simulink model "AutoTranscontrol"  (R2020a)
settings: Solver=VariableStepAuto  StartTime=0.0  StopTime=10.0  RelTol=1e-3
values from neighbouring files (symbols this model uses):
  N20 = 0    [matlab_workspace.mat]
  Rfd = 3.23    [matlab_workspace.mat]
  rload0 = 40    [matlab_workspace.mat]
  rload2 = 0.02    [matlab_workspace.mat]
undefined symbols (not defined in the file or in its folder): EMAP, Kfactor, NE_VEC, speedratio, TH_VEC, Torkratio
settings Model: Creator=DELL  LastModifiedBy=DELL

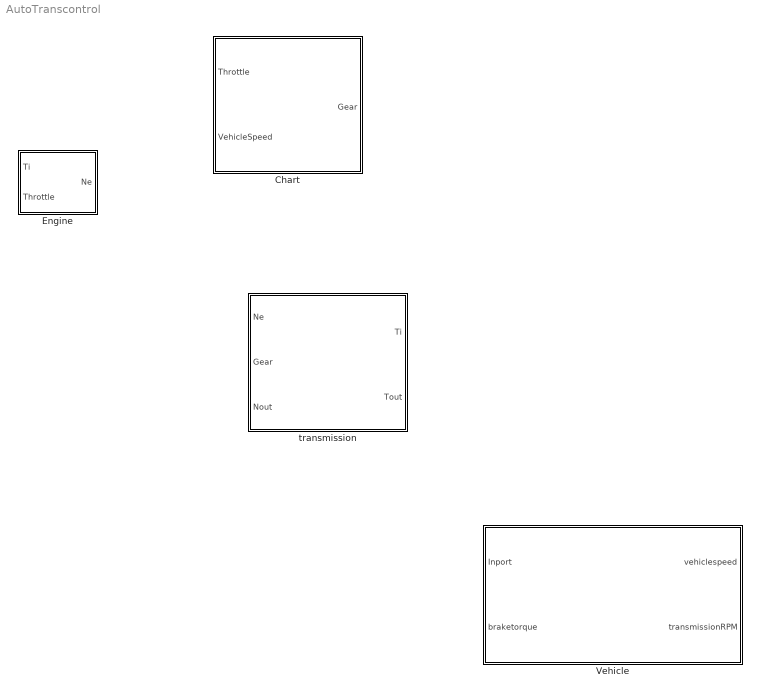
== system AutoTranscontrol ==
  Chart : Stateflow chart  TreatAsAtomicUnit=on
  Engine : Subsystem
  Vehicle : Subsystem
  transmission : Subsystem

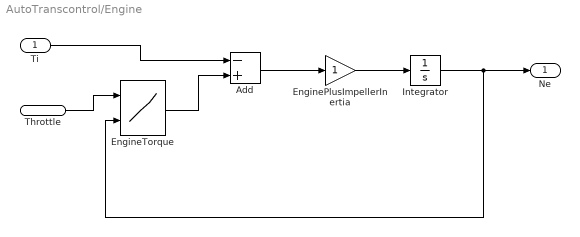
== system AutoTranscontrol/Engine ==
  Ti : Inport
  Throttle : Inport  Port=2
  Add : Sum  Inputs=-+
  EnginePlusImpellerInertia : Gain
  EngineTorque : Lookup_n-D  BreakpointsForDimension1=TH_VEC  BreakpointsForDimension2=NE_VEC  Table=EMAP  InputSameDT=on
  Integrator : Integrator  InitialCondition=1000  LimitOutput=on  UpperSaturationLimit=6000  LowerSaturationLimit=600
  Ne : Outport
  wires:
  EngineTorque/1 -> Add/2
  Add/1 -> EnginePlusImpellerInertia/1
  EnginePlusImpellerInertia/1 -> Integrator/1
  Integrator/1 -> Ne/1, EngineTorque/2
  Throttle/1 -> EngineTorque/1
  Ti/1 -> Add/1

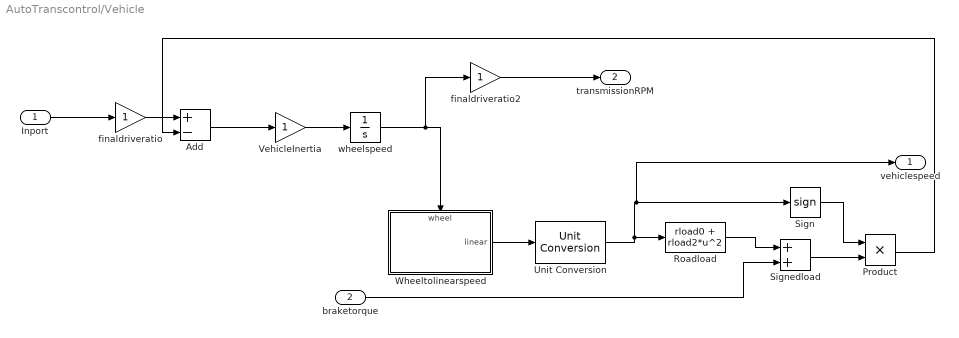
== system AutoTranscontrol/Vehicle ==
  Inport : Inport
  braketorque : Inport  Port=2
  Add : Sum  Inputs=+-
  Product : Product
  Roadload : Fcn  Expr=rload0 + rload2*u^2
  Sign : Signum
  Signedload : Sum
  Unit Conversion : UnitConversion
  VehicleInertia : Gain
  Wheeltolinearspeed : Subsystem
      settings: PortSchema="{\"entries\":[{\"content\":{\"sides\":[{\"content\":{\"connectorIds\":[]},\"type\":\"ConnectorPlacement.EquallySpacedRectSide\",\"uuid\":\"2d58122c-0a3c-46f5-9321-3a755b24d464\"},{\"content\":{\"connectorIds\":[\"Out1\"],\"side\":\"RIGHT\"},\"type\":\"ConnectorPlacement.EquallySpacedRectSide\",\"uuid\":\"52cb0b0a-ba8b-4201-a7b8-30d9f0796115\"},{\"content\":{\"connectorIds\":[\"In1\"],\"side\":\"TOP\"},\"type\":\"ConnectorPlacement.EquallySpacedRectSide\",\"uuid\":\"7f9df07b-7834-406d-9b53-00495da306c5\"}]},\"type\":\"ConnectorPlacement.EquallySpacedConnector\",\"uuid\":\"a8080389-0215-4d88-8d1d-d050e8a96295\"}],\"packageUris\":[\"http://schema.mathworks.com/mf0/Connector/19700101\"],\"version\":\"1.0\"}"
  finaldriveratio : Gain
  finaldriveratio2 : Gain
  wheelspeed : Integrator  InitialCondition=N20/Rfd
  vehiclespeed : Outport
  transmissionRPM : Outport  Port=2
  wires:
  wheelspeed/1 -> Wheeltolinearspeed/1(wheel), finaldriveratio2/1
  finaldriveratio/1 -> Add/1
  Inport/1 -> finaldriveratio/1
  Signedload/1 -> Product/2
  Sign/1 -> Product/1
  Wheeltolinearspeed/1(linear) -> Unit Conversion/1
  Add/1 -> VehicleInertia/1
  Roadload/1 -> Signedload/1
  Product/1 -> Add/2
  Unit Conversion/1 -> vehiclespeed/1, Sign/1, Roadload/1
  VehicleInertia/1 -> wheelspeed/1
  finaldriveratio2/1 -> transmissionRPM/1
  braketorque/1 -> Signedload/2

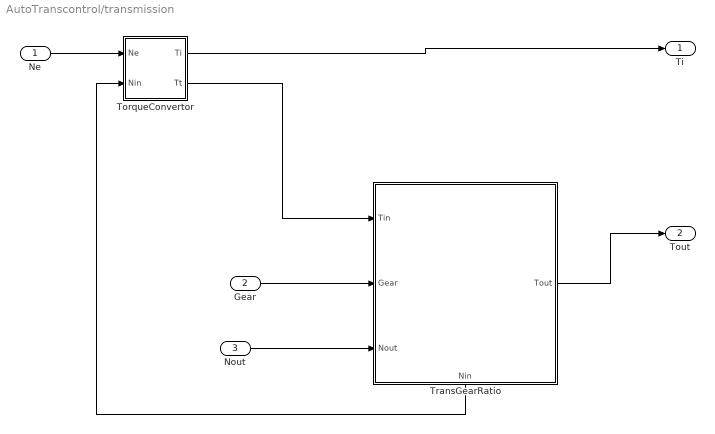
== system AutoTranscontrol/transmission ==
  Ne : Inport
  Gear : Inport  Port=2
  Nout : Inport  Port=3
  TorqueConvertor : Subsystem
  TransGearRatio : Subsystem
      settings: PortSchema="{\"entries\":[{\"content\":{\"sides\":[{\"content\":{\"connectorIds\":[\"In1\",\"In2\",\"In3\"]},\"type\":\"ConnectorPlacement.EquallySpacedRectSide\",\"uuid\":\"09106b39-6107-4922-852a-b097baa80348\"},{\"content\":{\"connectorIds\":[\"Out1\"],\"side\":\"RIGHT\"},\"type\":\"ConnectorPlacement.EquallySpacedRectSide\",\"uuid\":\"a36499d8-4a64-4af8-b2a6-947dde178184\"},{\"content\":{\"connectorIds\":[],\"side\":\"TOP\"},\"type\":\"ConnectorPlacement.EquallySpacedRectSide\",\"uuid\":\"0760f0ab-9b3f-4350-8835-7d8dce412455\"},{\"content\":{\"connectorIds\":[\"Out2\"],\"side\":\"BOTTOM\"},\"type\":\"ConnectorPlacement.EquallySpacedRectSide\",\"uuid\":\"6f573f33-3036-4647-848b-7112eae27f22\"}]},\"type\":\"ConnectorPlacement.EquallySpacedConnector\",\"uuid\":\"7220d938-930b-4b39-bb4b-0064243f33d7\"}],\"packageUris\":[\"http://schema.mathworks.com/mf0/Connector/19700101\"],\"version\":\"1.0\"}"
  Ti : Outport
  Tout : Outport  Port=2
  wires:
  Gear/1 -> TransGearRatio/2(Gear)
  Ne/1 -> TorqueConvertor/1(Ne)
  TorqueConvertor/1(Ti) -> Ti/1
  Nout/1 -> TransGearRatio/3(Nout)
  TransGearRatio/1(Tout) -> Tout/1
  TransGearRatio/2(Nin) -> TorqueConvertor/2(Nin)
  TorqueConvertor/2(Tt) -> TransGearRatio/1(Tin)

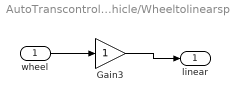
== system AutoTranscontrol/Vehicle/Wheeltolinearspeed ==
  wheel : Inport
  Gain3 : Gain
  linear : Outport
  wires:
  Gain3/1 -> linear/1
  wheel/1 -> Gain3/1

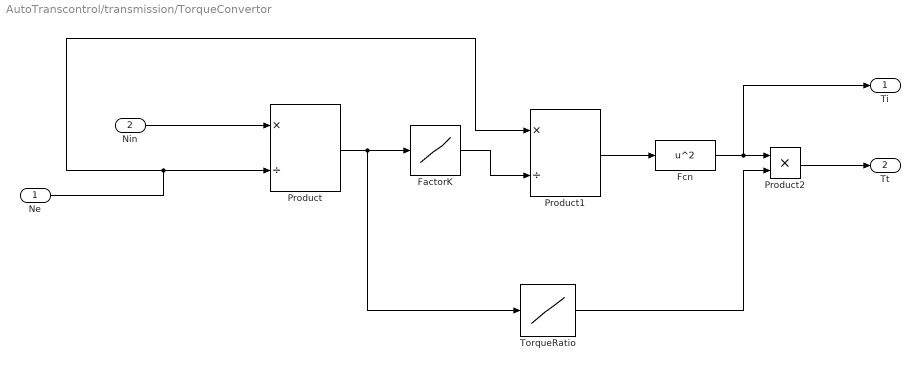
== system AutoTranscontrol/transmission/TorqueConvertor ==
  Ne : Inport
  Nin : Inport  Port=2
  FactorK : Lookup_n-D  NumberOfTableDimensions=1  BreakpointsForDimension1=speedratio  Table=Kfactor  SaturateOnIntegerOverflow=on  InputSameDT=on
  Fcn : Fcn  Expr=u^2
  Product : Product  Inputs=*/
  Product1 : Product  Inputs=*/
  Product2 : Product
  TorqueRatio : Lookup_n-D  NumberOfTableDimensions=1  BreakpointsForDimension1=speedratio  Table=Torkratio  SaturateOnIntegerOverflow=on  InputSameDT=on
  Ti : Outport
  Tt : Outport  Port=2
  wires:
  Product/1 -> TorqueRatio/1, FactorK/1
  Ne/1 -> Product1/1, Product/2
  FactorK/1 -> Product1/2
  Fcn/1 -> Ti/1, Product2/1
  Nin/1 -> Product/1
  Product2/1 -> Tt/1
  TorqueRatio/1 -> Product2/2
  Product1/1 -> Fcn/1

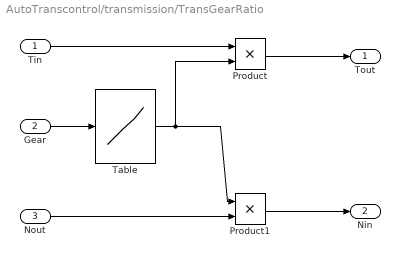
== system AutoTranscontrol/transmission/TransGearRatio ==
  Tin : Inport  Unit=ft*lbf@torque
  Gear : Inport  Port=2  Unit=1
  Nout : Inport  Port=3  Unit=rpm
  Product : Product  InputSameDT=on  SaturateOnIntegerOverflow=on  OutDataTypeStr=Inherit: Same as first input
  Product1 : Product  InputSameDT=on  SaturateOnIntegerOverflow=on  OutDataTypeStr=Inherit: Same as first input
  Table : Lookup_n-D  NumberOfTableDimensions=1  BreakpointsForDimension1=[1 2 3 4]  Table=[2.393 1.450 1.000 0.677]  OutDataTypeStr=double  SaturateOnIntegerOverflow=on  InputSameDT=on  LockScale=on
  Tout : Outport  Unit=ft*lbf@torque  VectorParamsAs1DForOutWhenUnconnected=off
  Nin : Outport  Port=2  Unit=rpm  VectorParamsAs1DForOutWhenUnconnected=off
  wires:
  Product1/1 -> Nin/1
  Table/1 -> Product1/1, Product/2
  Gear/1 -> Table/1
  Product/1 -> Tout/1
  Nout/1 -> Product1/2
  Tin/1 -> Product/1

== stateflow chart AutoTranscontrol/Chart ==
  state gearstate [parallel]
    settings: executionOrder=1
    state first
      entry:
      Gear=1;
    state second
      entry:
      Gear=2;
    state third
      entry:
      Gear=3;
    state fourth
      entry:
      Gear=4;
    (default) -> first
    first -> second : UP
    second -> third [order 1] : UP
    third -> fourth [order 1] : UP
    fourth -> third : DOWN
    third -> second [order 2] : DOWN
    second -> first [order 2] : DOWN
  state Selection [parallel]
    settings: executionOrder=2
    state steady_state
    state upshifting
    state downshifting
    (default) -> steady_state
    steady_state -> upshifting [order 1] : [VehicleSpeed > up_th]
    steady_state -> downshifting [order 2] : [VehicleSpeed < down_th]
    downshifting -> steady_state [order 1] : after(TWAIT,tick)
        | [VehicleSpeed <= down_th]
        | {DOWN}
    downshifting -> steady_state [order 2] : [VehicleSpeed > down_th]
    upshifting -> steady_state [order 1] : after(TWAIT,tick)
        | [VehicleSpeed >= up_th]
        | {UP}
    upshifting -> steady_state [order 2] : [VehicleSpeed < up_th]
  data: Throttle input; VehicleSpeed input; Gear output; TWAIT parameter; down_th local; up_th local
  events: UP local FUNCTION_CALL_EVENT; DOWN local FUNCTION_CALL_EVENT
